simulink model "bicycle_kinematic"  (R2025b)
settings: Solver=ode45  StartTime=0.0  StopTime=10.0  RelTol=1e-4
InitFcn:
  | run('init_vehicle_params.m')
values from neighbouring files (symbols this model uses):
  delta_max = deg2rad(27)    [init_vehicle_params.m]
  dmax_deg = 27.0    (= 27)    [init_vehicle_params.m]
  L = rosParams.wheel_base    [init_vehicle_params.m]    (also in vehi_param.m = 2 * (r + w * a_ratio) * sin(acos(1 - (s * w * a_ratio) / (r )
  Nc = Np    [AdaptiveLinMPC.m]    (also in init_vehicle_params.m = 3)
  Np = max(1, round(Np))    [AdaptiveLinMPC.m]    (also in init_vehicle_params.m = 10)
  Qpsi = max(Qpsi,   1e-4)    [AdaptiveLinMPC.m]    (also in init_vehicle_params.m = 1; mpc_cost_fun.m = x.Qpsi)
  Qy = max(Qy,     1e-4)    [AdaptiveLinMPC.m]    (also in init_vehicle_params.m = 1; mpc_cost_fun.m = x.Qy)
  R = Rdelta    [AdaptiveLinMPC.m]
  v0 = 3.0    (= 3)    [init_vehicle_params.m]
  vehicleParams = vehi_param(rosParams, tireParams, assumptions)    [init_vehicle_params.m]    (also in vehi_param.m = struct)
settings Model: Creator=yoo  LastModifiedBy=yoo
settings SolverCC: ZeroCrossControl=DisableAll

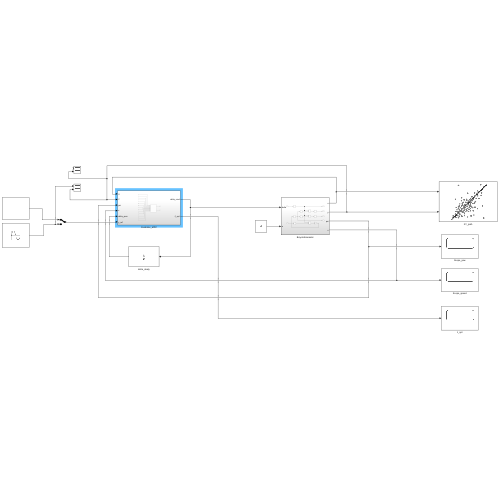
[thumbnail: Simulink's stored preview of the top-level diagram]
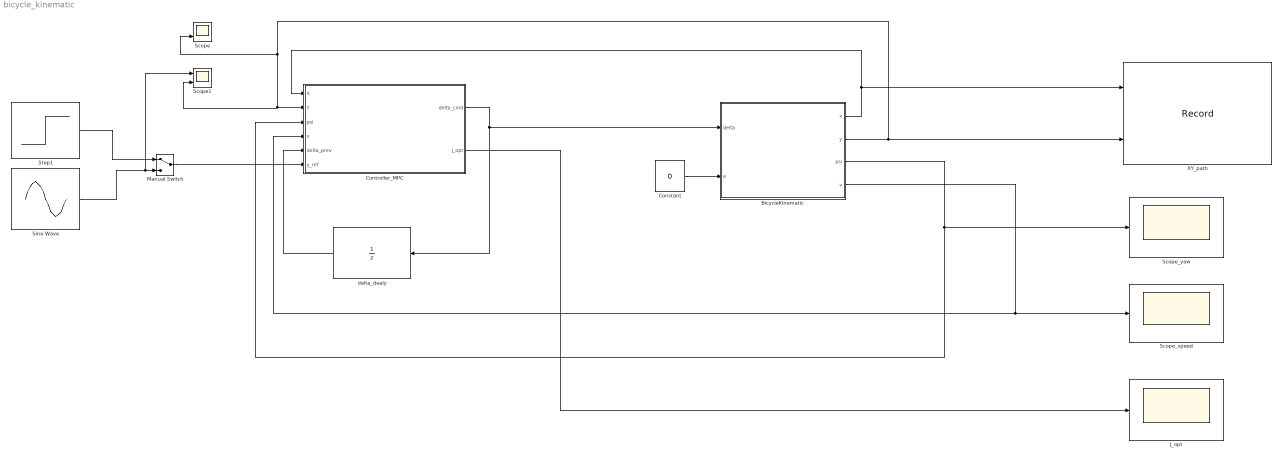
== system bicycle_kinematic ==
  BicycleKinematic : Subsystem
  Constant : Constant  Value=0
  Controller_MPC : Subsystem
  J_opt : Scope
      settings: ActiveDisplayYMinimum=-269.32940271572431  ActiveDisplayYMaximum=58.127890076972491  DataLoggingVariableName=ScopeData2
  Manual Switch : ManualSwitch
  Scope : Scope  NumInputPorts=2
      settings: ActiveDisplayYMinimum=-38.605203844181574  ActiveDisplayYMaximum=39.732140763012318  DataLoggingVariableName=ScopeData3
  Scope1 : Scope  NumInputPorts=2
      settings: ActiveDisplayYMinimum=-36.358713722341662  ActiveDisplayYMaximum=21.610517762723607  DataLoggingVariableName=ScopeData4
  Scope_speed : Scope
      settings: ActiveDisplayYMinimum=1.8747140250540708  ActiveDisplayYMaximum=13.127573774513367
  Scope_yaw : Scope
      settings: ActiveDisplayYMinimum=-11.523495026008819  ActiveDisplayYMaximum=13.771135680152755
  Sine Wave : Sin  SampleTime=0
  Step1 : Step  SampleTime=0
  XY_path : Record  NumPorts=2.0  FileSettingsInternal="{\"entries\":[{\"content\":{\"excelSettings\":{\"content\":{},\"type\":\"Streamout.ExcelSettings\"},\"parquetSettings\":{\"content\":{},\"type\":\"Streamout.ParquetSettings\"}},\"type\":\"Streamout.FileSettingStorage\",\"uuid\":\"\"}],\"packageUris\":[\"http:\\/\\/schema.mathworks.com\\/mf0\\/streamout_blocks\\/R2020a\"],\"version\":\"1.0\"}"  FrameSettings=[0, 0]  Layout=[1 1]  SignalsInternal="{\"entries\":[{\"content\":{\"signals\":[{\"content\":{\"blockPath\":[],\"dimensions\":[1],\"domain\":\"\",\"lineColor\":\"#a2142f\",\"plots\":[ 1 ],\"port\":1,\"sid\":[\"\"],\"signalID\":1,\"signalName\":\"BicycleKinematic:1\"},\"type\":\"RecordBlkView.Signal\",\"uuid\":\"\"},{\"content\":{\"blockPath\":[],\"dimensions\":[1],\"domain\":\"\",\"lineColor\":\"#139fff\",\"plots\":[ 1 ],\"port\":2,\"sid\":[\"\"],\"signalID\":2,\"signalName\":\"BicycleKinematic:2\"},\"type\":\"RecordBlkView.Signal\",\"uuid\":\"\"}]},\"type\":\"RecordBlkView.InputSignals\",\"uuid\":\"\"}],\"packageUris\":[\"http:\\/\\/schema.mathworks.com\\/mf0\\/streamout_blocks\\/R2020a\"],\"version\":\"1.0\"}"  VisualizationBindings="{\"xyplotplugin\":{\"info\":[{\"series\":[{\"bindingParametersList\":[{\"parameter\":\"X-Axis\",\"signalID\":1,\"signalName\":\"BicycleKinematic:1\"},{\"parameter\":\"Y-Axis\",\"signalID\":2,\"signalName\":\"BicycleKinematic:2\"}],\"seriesID\":0}],\"subplotID\":1}]}}"  CompatibilityTag=XY
  delta_dealy : UnitDelay  SampleTime=0.05  HasFrameUpgradeWarning=on
  wires:
  BicycleKinematic/2(y) -> Scope1/2, Controller_MPC/2(Y), Scope/2, XY_path/2
  BicycleKinematic/3(psi) -> Controller_MPC/3(psi), Scope_yaw/1
  BicycleKinematic/4(v) -> Controller_MPC/4(v), Scope_speed/1
  Controller_MPC/1(delta_cmd) -> BicycleKinematic/1(delta), delta_dealy/1
  delta_dealy/1 -> Controller_MPC/5(delta_prev)
  BicycleKinematic/1(x) -> Controller_MPC/1(X), XY_path/1
  Controller_MPC/2(J_opt) -> J_opt/1
  Sine Wave/1 -> Scope1/1, Manual Switch/2
  Manual Switch/1 -> Controller_MPC/6(y_ref)
  Constant/1 -> BicycleKinematic/2(a)
  Step1/1 -> Manual Switch/1

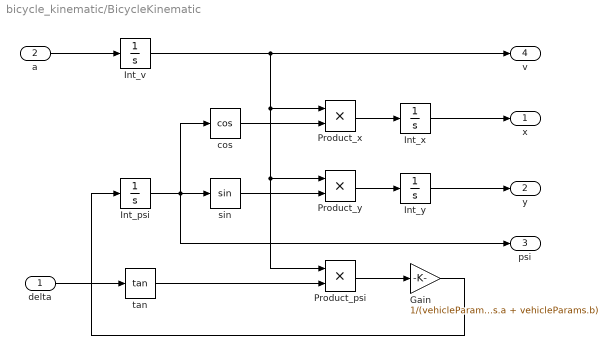
== system bicycle_kinematic/BicycleKinematic ==
  delta : Inport
  a : Inport  Port=2
  Gain : Gain  Gain=1/(vehicleParams.a + vehicleParams.b)
  Int_psi : Integrator
  Int_v : Integrator  InitialCondition=v0
  Int_x : Integrator
  Int_y : Integrator
  Product_psi : Product
  Product_x : Product
  Product_y : Product
  cos : Trigonometry  Operator=cos
  sin : Trigonometry
  tan : Trigonometry  Operator=tan
  x : Outport
  y : Outport  Port=2
  psi : Outport  Port=3
  v : Outport  Port=4
  wires:
  delta/1 -> tan/1
  Int_psi/1 -> cos/1, sin/1, psi/1
  Int_v/1 -> v/1, Product_psi/1, Product_y/1, Product_x/1
  cos/1 -> Product_x/2
  Product_x/1 -> Int_x/1
  sin/1 -> Product_y/2
  Product_y/1 -> Int_y/1
  tan/1 -> Product_psi/2
  a/1 -> Int_v/1
  Product_psi/1 -> Gain/1
  Gain/1 -> Int_psi/1
  Int_x/1 -> x/1
  Int_y/1 -> y/1

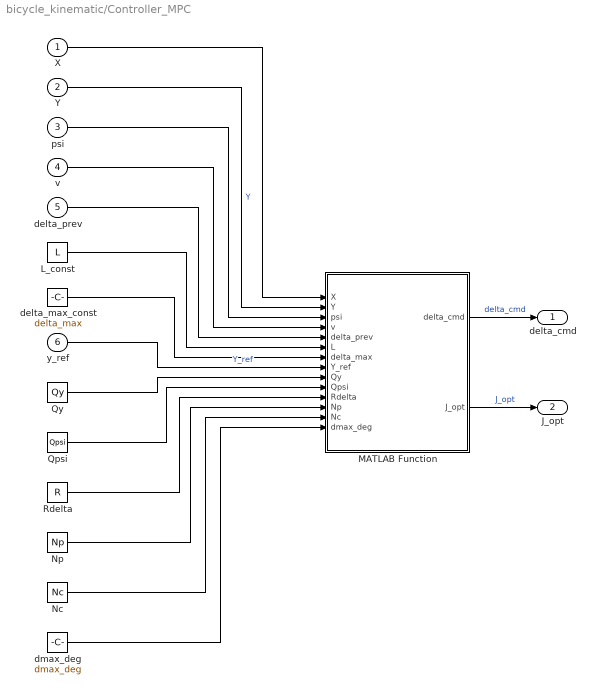
== system bicycle_kinematic/Controller_MPC ==
  X : Inport
  Y : Inport  Port=2
  psi : Inport  Port=3
  v : Inport  Port=4
  delta_prev : Inport  Port=5
  y_ref : Inport  Port=6
  L_const : Constant  Value=L
  MATLAB Function : MATLAB Function  TreatAsAtomicUnit=on
  Nc : Constant  Value=Nc
  Np : Constant  Value=Np
  Qpsi : Constant  Value=Qpsi
  Qy : Constant  Value=Qy
  Rdelta : Constant  Value=R
  delta_max_const : Constant  Value=delta_max
  dmax_deg : Constant  Value=dmax_deg
  delta_cmd : Outport
  J_opt : Outport  Port=2
  wires:
  X/1 -> MATLAB Function/1(X)
  Y/1 -> MATLAB Function/2(Y)  "Y"
  psi/1 -> MATLAB Function/3(psi)
  v/1 -> MATLAB Function/4(v)
  delta_prev/1 -> MATLAB Function/5(delta_prev)
  MATLAB Function/1(delta_cmd) -> delta_cmd/1  "delta_cmd"
  L_const/1 -> MATLAB Function/6(L)
  delta_max_const/1 -> MATLAB Function/7(delta_max)
  MATLAB Function/2(J_opt) -> J_opt/1  "J_opt"
  y_ref/1 -> MATLAB Function/8(Y_ref)  "Y_ref"
  Qy/1 -> MATLAB Function/9(Qy)
  Qpsi/1 -> MATLAB Function/10(Qpsi)
  Rdelta/1 -> MATLAB Function/11(Rdelta)
  Np/1 -> MATLAB Function/12(Np)
  Nc/1 -> MATLAB Function/13(Nc)
  dmax_deg/1 -> MATLAB Function/14(dmax_deg)

== matlab function bicycle_kinematic/Controller_MPC/MATLAB Function ==
  data: X input; delta_cmd output; Y input; psi input; v input; delta_prev input; L input; delta_max input; J_opt output; Y_ref input; Qy input; Qpsi input; Rdelta input; Np input; Nc input; dmax_deg input
function [delta_cmd, J_opt] = AdaptiveLinMPC( ...
    X, Y, psi, v, delta_prev, ...
    L, delta_max, Y_ref, ...
    Qy, Qpsi, Rdelta, Np, Nc, dmax_deg)
%#codegen
% Adaptive linear MPC based on linearized kinematic bicycle model
% - Vehicle params (L, delta_max)는 Simulink Constant 블록에서 입력
% - MPC params (Qy, Qpsi, Rdelta, Np, Nc, dmax_deg)는 외부에서 튜닝/최적화

    %----- 외부 QP 솔버 선언 (코드 생성 대상 아님) -----
    coder.extrinsic('quadprog','optimoptions');

    %----- 기본 출력값 -----
    delta_cmd = delta_prev;    % 실패 시 이전 조향 유지
    J_opt     = NaN;           % 최적비용 기본값 (해를 못 찾으면 NaN)

    %================== 0) 파라미터 방어 코드 ==================    
    Ts = 0.05;                 % 샘플링 타임 (고정)

    % horizon 방어: 0, 음수, Nc> Np 방지
    Np = max(1, round(Np));
    Nc = max(1, round(Nc));
    if Nc > Np
        Nc = Np;
    end

    % 가중치 하한 (너무 작아서 H가 singular 되는 것 방지)
    Qy     = max(Qy,     1e-4);
    Qpsi   = max(Qpsi,   1e-4);
    Rdelta = max(Rdelta, 1e-5);

    % Q 구성 (X, v는 0, Y/psi만 튜닝)
    Q = diag([0, Qy, Qpsi, 0]);

    % R (스칼라)
    R = Rdelta;

    % Δδ (스텝당 조향 변화량) 제약 [rad]
    d_step_max = dmax_deg * pi/180.0;    % 입력은 deg → rad
    d_step_max = max(d_step_max, 0.5*pi/180.0);  % 최소 약 0.5deg
    lb = -d_step_max * ones(Nc,1);
    ub =  d_step_max * ones(Nc,1);

    % 절대 조향 한계 (rad) – 입력 delta_max 사용
    delta_limit = abs(delta_max);
    if delta_limit <= 0
        delta_limit = 30*pi/180.0;       % 비정상 값이면 30deg 기본
    end
    delta_min = -delta_limit;
    delta_max_abs =  delta_limit;

    %================== 1) 현재 상태 주변에서 선형화 (A,B) ==================
    % 비선형 모델
    %  dot X   = v*cos(psi)
    %  dot Y   = v*sin(psi)
    %  dot psi = (v/L)*tan(delta)
    %  dot v   = a

    % 수치 안정용: v가 너무 작으면 최소값
    v_lin = max(v, 0.1);

    A = [ 0, 0, -v_lin*sin(psi),  cos(psi);
          0, 0,  v_lin*cos(psi),  sin(psi);
          0, 0,  0,               (1/L)*tan(delta_prev);
          0, 0,  0,               0 ];

    B = [ 0;
          0;
          (v_lin/L)*sec(delta_prev)^2;
          0 ];

    %================== 2) 이산화 (Forward Euler) ==================
    Ad = eye(4) + Ts*A;
    Bd = Ts * B;

    %================== 3) MPC 설정 ==================
    % 상태벡터: x = [X; Y; psi; v]
    xk = [X; Y; psi; v];

    % 간단한 레인-중심/헤딩 제어:
    X_ref   = X;        % 종방향은 그대로
    psi_ref = 0;
    v_ref   = v;
    
    xref = [X_ref; Y_ref; psi_ref; v_ref];    % Y_ref는 입력
    xt   = xk - xref;                         % 편차 상태

    % Prediction matrices
    [Phi, Gamma] = build_prediction_matrices(Ad, Bd, Np, Nc);

    Qbar = kron(eye(Np), Q);
    Rbar = kron(eye(Nc), R);

    %================== 4) QP 행렬 H, f 구성 ==================
    % 예측: X_stack = Phi*xt + Gamma*dU
    % 비용: J = X'QbarX + dU'Rbar dU
    H = Gamma' * Qbar * Gamma + Rbar;
    f = Gamma' * Qbar * (Phi * xt);

    % 수치 안정성용 대칭화 + regularization
    H = (H + H')/2;
    H = H + 1e-8*eye(size(H));

    %================== 5) quadprog 호출 ==================
    dU    = zeros(Nc,1);    % 기본값: 변화 없음
    J_opt = NaN;            % 기본값: 비용 미정

    % H, f가 비어 있거나 차원이 0이면 QP 풀지 않음
    if ~isempty(H) && ~isempty(f)
        nvar = length(f);
        if nvar > 0
            opts = optimoptions('quadprog','Display','off');
            % extrinsic → dU_sol, fval, exitflag는 mxArray로 넘어옴
            [dU_sol, fval, exitflag] = quadprog(H, f, [], [], [], [], lb, ub, [], opts);

            % extrinsic 출력은 mxArray지만, isempty(dU_sol)는 허용되는 패턴
            if ~isempty(dU_sol)
                dU    = dU_sol;
                J_opt = fval;
            else
                % 해를 못 찾으면 dU는 0 유지, J_opt는 NaN
                J_opt = NaN;
            end
        end
    end

    %================== 6) 최종 조향 명령 (클램프 포함) ==================
    delta_raw = delta_prev + dU(1);

    % 절대 조향 한계 적용
    delta_cmd = min(max(delta_raw, delta_min), delta_max_abs);
end


%====================================================================
% 로컬 함수: Prediction matrices Phi, Gamma 생성
%====================================================================
function [Phi, Gamma] = build_prediction_matrices(Ad, Bd, Np, Nc)

    n = size(Ad,1);   % 상태 차원 (4)
    m = size(Bd,2);   % 입력 차원 (조향 하나라고 가정하지만 일반화)

    Phi   = zeros(Np*n, n);
    Gamma = zeros(Np*n, Nc*m);

    %----- Phi 계산: A, A^2, ..., A^Np -----
    A_power = eye(n);
    for i = 1:Np
        A_power = Ad * A_power;
        Phi((i-1)*n+1:i*n, :) = A_power;
    end

    %----- Gamma 계산: Toeplitz 형태 -----
    for r = 1:Np
        for c = 1:Nc
            if r >= c
                % Ad^(r-c) * Bd
                A_pc = eye(n);
                for k = 1:(r-c)
                    A_pc = Ad * A_pc;
                end
                Gamma((r-1)*n+1:r*n, (c-1)*m+1:c*m) = A_pc * Bd;
            end
        end
    end
end
